simulink model "simulink_cascade22"  (R2023a)
settings: Solver=ode4  StartTime=0.0  StopTime=20  FixedStep=0.001  RelTol=1e-3
values from neighbouring files (symbols this model uses):
  G = tf(modello_continuo_g1_3rd)    [simulink_config.m]
undefined symbols (not defined in the file or in its folder): Ki1_vel, Kp1_pos, Kp1_vel, Tf1_pos, Tf1_vel, Wn_notch1, xci_p1, xci_z1
libraries: simulink x4
settings Model: Creator=edoar  LastModifiedBy=edoar
settings SolverCC: AlgebraicLoopSolver=TrustRegion
settings DebuggingCC: UnconnectedInputMsg=warning  UnconnectedOutputMsg=warning  UnconnectedLineMsg=warning
settings ModelReferenceCC: EnableRefExpFcnMdlSchedulingChecks=on

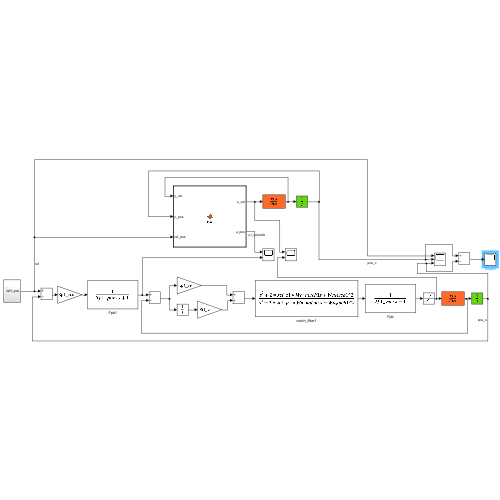
[thumbnail: Simulink's stored preview of the top-level diagram]
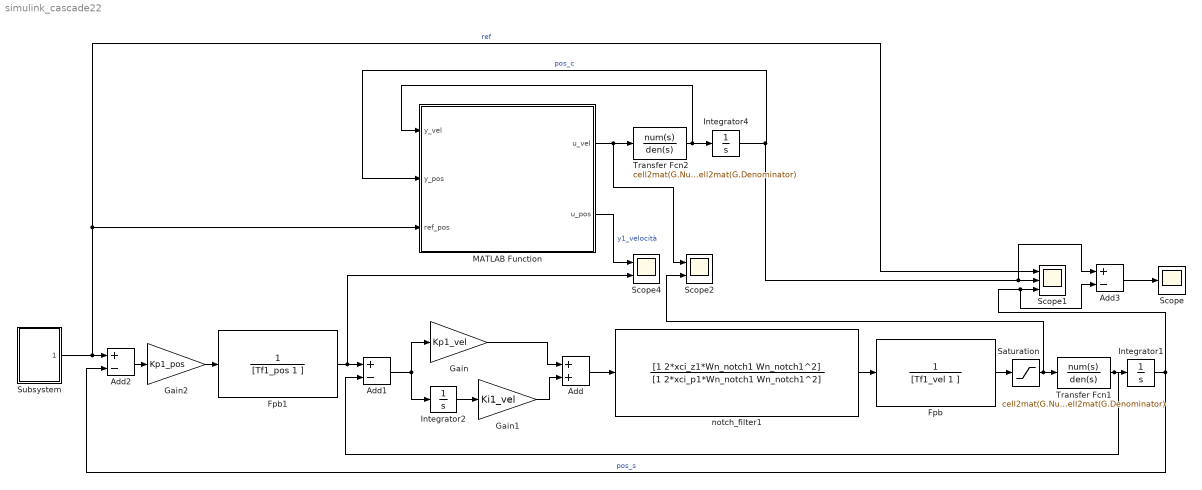
== system simulink_cascade22 ==
  Add : Sum
  Add1 : Sum  Inputs=+-
  Add2 : Sum  Inputs=+-
  Add3 : Sum  Inputs=+-
  Fpb : TransferFcn  Numerator=1  Denominator=[Tf1_vel 1 ]
  Fpb1 : TransferFcn  Numerator=1  Denominator=[Tf1_pos 1 ]
  Gain : Gain  Gain=Kp1_vel
  Gain1 : Gain  Gain=Ki1_vel
  Gain2 : Gain  Gain=Kp1_pos
  Integrator1 : Integrator
  Integrator2 : Integrator
  Integrator4 : Integrator
  MATLAB Function : MATLAB Function  TreatAsAtomicUnit=on
  Saturation : Saturate  UpperLimit=600  LowerLimit=-600
  Scope : Scope
  Scope1 : Scope  NumInputPorts=3
  Scope2 : Scope  NumInputPorts=2
  Scope4 : Scope  NumInputPorts=2
  Subsystem : Subsystem
  Transfer Fcn1 : TransferFcn  Numerator=cell2mat(G.Numerator)  Denominator=cell2mat(G.Denominator)
  Transfer Fcn2 : TransferFcn  Numerator=cell2mat(G.Numerator)  Denominator=cell2mat(G.Denominator)
  notch_filter1 : TransferFcn  Numerator=[1 2*xci_z1*Wn_notch1 Wn_notch1^2]  Denominator=[1 2*xci_p1*Wn_notch1 Wn_notch1^2]
  wires:
  Gain1/1 -> Add/2
  Add1/1 -> Gain/1, Integrator2/1
  Saturation/1 -> Scope2/2, Transfer Fcn1/1
  Add2/1 -> Gain2/1
  Add/1 -> notch_filter1/1
  notch_filter1/1 -> Fpb/1
  Gain/1 -> Add/1
  Integrator1/1 -> Scope1/3, Add3/2, Add2/2  "pos_s"
  Gain2/1 -> Fpb1/1
  Fpb1/1 -> Scope4/2, Add1/1
  Integrator4/1 -> Add3/1, Scope1/2, MATLAB Function/2(y_pos)  "pos_c"
  Fpb/1 -> Saturation/1
  Transfer Fcn1/1 -> Add1/2, Integrator1/1
  Integrator2/1 -> Gain1/1
  MATLAB Function/1(u_vel) -> Scope2/1, Transfer Fcn2/1
  MATLAB Function/2(u_pos) -> Scope4/1  "y1_velocità"
  Subsystem/1(ref1_pos) -> MATLAB Function/3(ref_pos), Scope1/1, Add2/1  "ref"
  Transfer Fcn2/1 -> Integrator4/1, MATLAB Function/1(y_vel)
  Add3/1 -> Scope/1

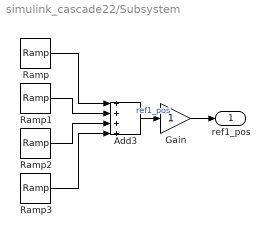
== system simulink_cascade22/Subsystem ==
  Add3 : Sum  Inputs=++++
  Gain : Gain
  Ramp : simulink/Sources/Ramp  slope=0.2  start=0  InitialOutput=0
  Ramp1 : simulink/Sources/Ramp  slope=-0.2  start=5  InitialOutput=0
  Ramp2 : simulink/Sources/Ramp  slope=-0.2  start=10  InitialOutput=0
  Ramp3 : simulink/Sources/Ramp  slope=0.2  start=15  InitialOutput=0
  ref1_pos : Outport
  wires:
  Ramp1/1 -> Add3/2
  Ramp/1 -> Add3/1
  Ramp2/1 -> Add3/3
  Add3/1 -> Gain/1  "ref1_pos"
  Ramp3/1 -> Add3/4
  Gain/1 -> ref1_pos/1

== matlab function simulink_cascade22/MATLAB Function ==
  settings: updateMethod=DISCRETE
  data: y_vel input; y_pos input; ref_pos input; u_vel output; u_pos output
function [u_vel,u_pos] = fcn(y_vel,y_pos,ref_pos)
st = 0.001;
Kp_pos = 1.497822658004661e+02;
Kp_vel = 3.319250421479281e+03;
Ki_vel  = 1.770266891455617e+04;
Kaw = 5.93334;
UMax = 600;
%low pass filter esterno
nup_fpb =0.5;
num1p_fpb =0.5;
nym1p_fpb =0;
nyp_fpb =1;
%notch filter
nu_fn =0.765;
num1_fn =-1.111;
num2_fn =0.6368;
ny_fn =1;
nym1_fn =-1.111;
nym2_fn =0.4019;

%low pass filter esterno
nu_fpb=0.5;
num1_fpb=0.5;
nym1_fpb=0;
ny_fpb=1;

persistent a um2 um1 um2_notch um1_notch um1_pb xi um1p_pb

if isempty(a)
    a = 0;
    um2 = 0;
    um1 = 0;
    um2_notch=0;
    um1_notch=0;
    um1_pb=0;
    xi=0;
    um1p_pb=0;
    y_pos=0;
    y_vel=0;
end

%calcolo azione esterna
error_pos = ref_pos - y_pos;
%calcolo della azione di controllo del PI
u_now1 = Kp_pos*error_pos;
% applicazione filtro passa-basso
u_pos = ( nup_fpb*u_now1 +  num1p_fpb.*a -  nym1p_fpb* um1p_pb)/ nyp_fpb;

a = u_now1;   %u(t-1) = u_now
um1p_pb = u_pos;

%calcolo errore in ingresso al PI
error_vel = u_pos - y_vel;
%calcolo della azione di controllo del PI
u_now =  xi +  Kp_vel*error_vel;
% applicazione filtro notch
unotch = ( nu_fn*u_now +  num1_fn* um1 +  num2_fn* um2 -  nym1_fn* um1_notch -  nym2_fn* um2_notch)/ ny_fn;
%unotch=u_now;
% applicazione filtro passa-basso
un = ( nu_fpb*unotch +  num1_fpb* um1_notch -  nym1_fpb* um1_pb)/ ny_fpb;
    
if (un >  UMax) %saturazione positiva
    xi =  xi +  Ki_vel*error_vel*st +  Kaw*st*(UMax-un);
    un =  UMax;
elseif (un < - UMax) %saturazione negativa
    xi =  xi +  Ki_vel*error_vel*st +  Kaw*st*(-UMax-un);
    un = - UMax;
else % assenza saturazione
    xi =  xi +  Ki_vel*error_vel* st;
end

um2 = um1; %u(t-2) = u(t-1)
um1 = u_now;   %u(t-1) = u_now
um2_notch = um1_notch;
um1_notch = unotch;
um1_pb = un;

u_vel = un;
